simulink model "part7_modebutton_v2"  (R2022b)
settings: Solver=FixedStepAuto  StartTime=0.0  StopTime=100  FixedStep=0.01  RelTol=1e-3
libraries: simulink x3
settings Model: PacingRate=0.890000  Creator=mingreico  LastModifiedBy=mingreico

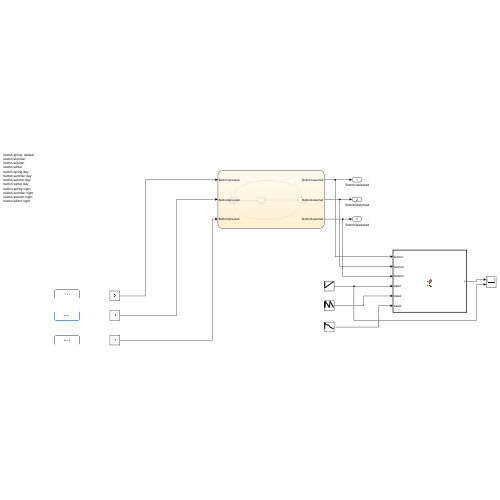
[thumbnail: Simulink's stored preview of the top-level diagram]
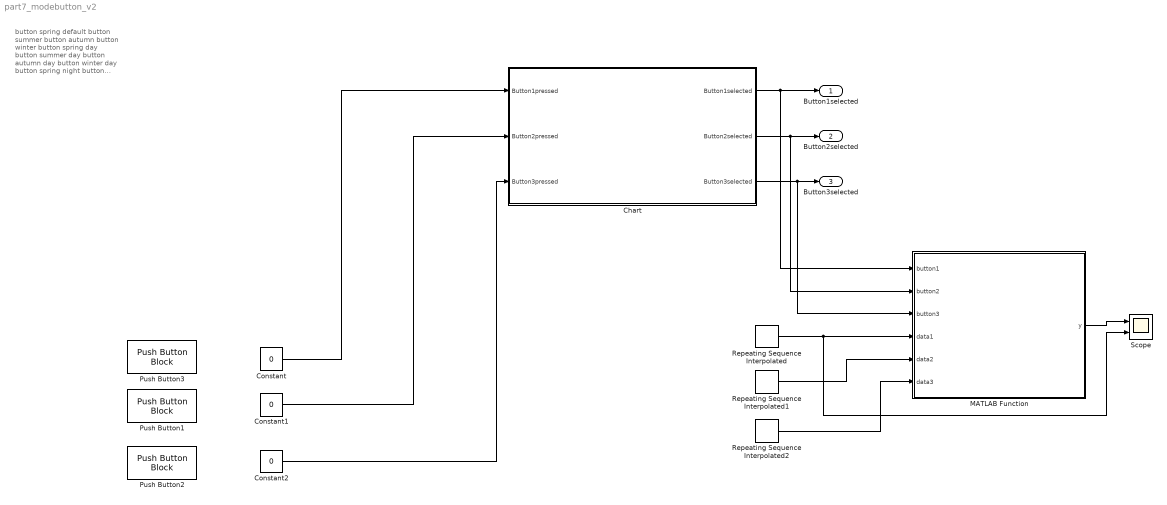
== system part7_modebutton_v2 ==
  note: button spring  default
      | button summer
      | button autumn
      | button winter
      | button spring day
      | button summer day
      | button autumn day
      | button winter day
      | button spring night
      | button summer night
      | button autumn night
      | button winter night
  Chart : Stateflow chart  TreatAsAtomicUnit=on
  Constant : Constant  Value=0  OutDataTypeStr=boolean
  Constant1 : Constant  Value=0  OutDataTypeStr=boolean
  Constant2 : Constant  Value=0  OutDataTypeStr=boolean
  MATLAB Function : MATLAB Function  TreatAsAtomicUnit=on
  Push Button1 : PushButtonBlock  ButtonText=Button2  OffValue=0.000000
  Push Button2 : PushButtonBlock  ButtonText=Button3  OffValue=0.000000
  Push Button3 : PushButtonBlock  ButtonText=Button1  OffValue=0.000000
  Repeating Sequence Interpolated : simulink/Sources/Repeating Sequence Interpolated  OutValues=[1 2 3 4 5].'  TimeValues=[0 1 2 3 4].'  LookUpMeth=Interpolation-Use End Values  tsamp=0.01  OutMin=[]  OutMax=[]  OutDataTypeStr=double  OutputDataTypeScalingMode=double  OutDataType=fixdt(0,8)  OutScaling=2^-10
  Repeating Sequence Interpolated1 : simulink/Sources/Repeating Sequence Interpolated  OutValues=[1 2 1 2 1].'  TimeValues=[0 0.1 0.5 0.6 1].'  LookUpMeth=Interpolation-Use End Values  tsamp=0.01  OutMin=[]  OutMax=[]  OutDataTypeStr=double  OutputDataTypeScalingMode=double  OutDataType=fixdt(0,8)  OutScaling=2^-10
  Repeating Sequence Interpolated2 : simulink/Sources/Repeating Sequence Interpolated  OutValues=[5 4 3 2 1].'  TimeValues=[0 0.1 0.5 0.6 1].'  LookUpMeth=Interpolation-Use End Values  tsamp=0.01  OutMin=[]  OutMax=[]  OutDataTypeStr=double  OutputDataTypeScalingMode=double  OutDataType=fixdt(0,8)  OutScaling=2^-10
  Scope : Scope  NumInputPorts=2
  " Button1selected" : Outport
  " Button2selected" : Outport  Port=2
  " Button3selected" : Outport  Port=3
  wires:
  Constant/1 -> Chart/1(Button1pressed)
  Constant1/1 -> Chart/2(Button2pressed)
  Constant2/1 -> Chart/3(Button3pressed)
  Chart/1(" Button1selected") -> MATLAB Function/1(button1), " Button1selected"/1
  Chart/2(" Button2selected") -> MATLAB Function/2(button2), " Button2selected"/1
  Chart/3(" Button3selected") -> " Button3selected"/1, MATLAB Function/3(button3)
  Repeating Sequence Interpolated/1 -> Scope/2, MATLAB Function/4(data1)
  Repeating Sequence Interpolated1/1 -> MATLAB Function/5(data2)
  Repeating Sequence Interpolated2/1 -> MATLAB Function/6(data3)
  MATLAB Function/1(y) -> Scope/1

== matlab function part7_modebutton_v2/MATLAB Function ==
  data: button1 input; button2 input; button3 input; data1 input; data2 input; y output; data3 input
function y = fcn(button1, button2, button3, data1,data2,data3)
    if button1
        y = data1;
    elseif button2
        y =data2;
    elseif button3
        y = data3;
    else 
        y = data1;
    end
end

== stateflow chart part7_modebutton_v2/Chart ==
  settings: executeAtInitialization=1
  state Button1selected
  state Button2selected
  state Button3selected
  Button1selected -> Button3selected [order 3] : [Button3pressed]
  (default) -> Button1selected
  Button2selected -> Button3selected [order 2] : [Button3pressed]
  Button1selected -> Button1selected [order 2] : [Button1pressed]
  Button3selected -> Button2selected [order 1] : [Button2pressed]
  Button1selected -> Button2selected [order 1] : [Button2pressed]
  Button2selected -> Button1selected [order 1] : [Button1pressed]
  Button3selected -> Button3selected [order 2] : [Button3pressed]
  Button3selected -> Button1selected [order 3] : [Button1pressed]
  Button2selected -> Button2selected [order 3] : [Button2pressed]
  data: Button1selected output boolean; Button2selected output boolean; Button3selected output boolean; Button1pressed input boolean size=1; Button2pressed input boolean size=1; Button3pressed input boolean size=1
